simulink model "RBFNN_1221"  (R2018a)
settings: Solver=FixedStepAuto  StartTime=0.0  StopTime=inf  FixedStep=0.001  RelTol=1e-3  EnableMultiTasking=on
undefined symbols (not defined in the file): HIL, j, qc_get_step_size
libraries: dsparch4 x28, quarc_library x17, simulink x7, vrlib x1
(part 5 of 6)

== matlab function RBFNN_1221/DIARC_new ==
  data: U output; mode_IARC input; switch_NN input; RBFNN input; qd input; qd_dot input; qd_ddot input; qd_dddot input; q input; q_dot input; P_i input; P_o input; P_s input; P_r input; K_1 input; K_2 input; K_3 input; w2 input; w3 input; gamma_d1 input; gamma_d2 input; vartheta_s1 input; vartheta_s2 input; d1hat input; d2hat input; Gamma1_1 input; Gamma1_2 input; Gamma1_3 input; Gamma1_4 input; Gamma2 input; X1_f input; q_ddot input; e2 output; e3 output; vartheta_s1_next output; vartheta_s2_next output; d1hat_next output; d2hat_next output; Gamma1_1_next output; Gamma1_2_next output; Gamma1_3_next output; Gamma1_4_next output; Gamma2_next output; X1f_next output; tolook_FLd output; tolook_QLd output; tolook_others output; tolook_FLda1_joint3 output
function [U, e2, e3, vartheta_s1_next, vartheta_s2_next, d1hat_next, d2hat_next,...
    Gamma1_1_next, Gamma1_2_next, Gamma1_3_next, Gamma1_4_next, Gamma2_next, X1f_next, ...
    tolook_FLd, tolook_QLd, tolook_others,tolook_FLda1_joint3] ...
    = DIARC_new(mode_IARC, switch_NN, RBFNN, qd, qd_dot, qd_ddot, qd_dddot, q, q_dot,...
    P_i, P_o, P_s, P_r, K_1, K_2, K_3, w2, w3, gamma_d1, gamma_d2,...
    vartheta_s1, vartheta_s2, d1hat, d2hat, Gamma1_1, Gamma1_2, Gamma1_3, Gamma1_4, Gamma2, X1_f,  q_ddot)
% --------------------------程序说明---------------------------
%
% Aunthor: Yangxiu Xia
% multi-DOF 关节空间主控程序，1.0版本完成时间
%
% --------------------------输入参数---------------------------
%
%      传感器部分
% qd:           R4*1，弧度制rad，分别为J1-J4的四个期望角度
% qd_dot:       R4*1，弧度制rad，分别为J1-J4的四个期望角速度
% qd_ddot:      R4*1，弧度制rad，分别为J1-J4的四个期望角加速度
% qd_dddot:     R4*1，弧度制rad，分别为J1-J4的四个期望角加加速度
% q:            R4*1，弧度制rad，分别为J1-J4的四个实际角度
% q_dot:        R4*1，弧度制rad，分别为J1-J4的四个实际角速度，通过前置快速微分滤波得到
% P_i:          R4*1，Pa，无杆腔压力
% P_o:          R4*1，Pa，有杆腔压力
% P_s:          R1*1，Pa，泵出压力
% P_r:          R1*1，Pa，油箱参考压力
%       控制部分
% K_1:          R4*1，(使用时是diag形式)，滑模增益，
% K_2:          R4*1，(使用时是diag形式)，step1线性反馈增益
% K_3:          R4*1，(使用时是diag形式)，step2线性反馈增益
% w2:           R4*1，(使用时是diag形式)，量纲平衡系数2
% w3:           R4*1，(使用时是diag形式)，量纲平衡系数336.
% gamma_d1:     R4*1，(使用时是diag形式)，step1快速动力学补偿项的更新增益
% gamma_d2:     R4*1，(使用时是diag形式)，step2快速动力学补偿项的更新增益
% vartheta_s1:  R12*1，[f_v, f_c, D_Fn] = [4个关节的粘性摩擦, 4个关节的库伦摩擦, 4个关节的建模误差名义值]
% vartheta_s2:  R9*1， [D_Qin, D_Qon, 1/Beta_e] = [4个关节的建模误差名义值1, 4个关节的建模误差名义值2，油液弹性模量]
% d1hat:        R4*1，step1快速动力学补偿项
% d2hat:        R4*1，step2快速动力学补偿项
% Gamma1:       R12*12，自适应律增益矩阵1
% Gamma2:       R9*9，  自适应律增益矩阵2
% X_f:          R37*1,  滤波中间量 = [vartheta_s1(12，无mL), u_s1f_A(4), pF(4), vartheta_s2(9), u_s2(4), pQ(4)]
% 
% --------------------------变量维度---------------------------
%
% M0:           R4*4，（不考虑负载）机械臂本体的惯性矩阵
% C0:           R4*4，（不考虑负载）机械臂本体的离心力与科氏力矩阵
% G0:           R4*1，（不考虑负载）机械臂本体的重力矩阵
% ML:           R4*4，负载带来的额外惯性矩阵
% CL:           R4*4，负载带来的额外离心力与科氏力矩阵
% GL:           R4*1，负载带来的额外重力矩阵
% alpha_DH:     R4*1，弧度制rad，控制三角形夹角
% q_ddot:       R4*1，弧度制rad，分别为J1-J4的四个实际角加速度
% q_dddot:      R4*1，弧度制rad，分别为J1-J4的四个实际角加加速度
% tau:          R4*1，机械臂驱动力矩，包括液压缸推力与摩擦
% D_Fn:         R4*1，机械臂刚体动力学的集总建模误差名义值
% D_Qin:        R4*1，容腔压力动力学的集总建模误差1名义值
% D_Qon:        R4*1，容腔压力动力学的集总建模误差2名义值
% J_h:          R4*4，非奇异关节雅各比矩阵
% F_L:          R4*1，液压缸输出推力
% T_f:          R4*1，摩擦力矩
% f_v:          R4*1，粘性摩擦系数 
% f_c:          R4*1，库伦摩擦系数
% A_o:          R4*4，有杆腔活塞面积
% V_i:          R4*4，无杆腔可压缩容积
% V_o:          R4*4，有杆腔可压缩容积
% x_L:          R4*1，液压缸位移
% Beta_e:       R1*1，油液弹性膜模量
% Q_i:          R4*1，无杆腔供应流量
% Q_o:          R4*1，有杆腔供应流量
% K_qi:         R4*1，无杆腔阀口流量增益系数
% K_qo:         R4*1，有杆腔阀口流量增益系数
% h_i:          R4*1，无杆腔压差
% A_i:          R4*4，无杆腔活塞面积
% h_o:          R4*1，有杆腔压差
% 
% -------------------------------------------------------------

%%
%-------输入模拟（维度范例）--------
% mode_mL = 1;
% qd = [1 2 3 4]'/57;
% qd_dot = [1 2 3 4]'/57;
% qd_ddot = [1 2 3 4]'/57;
% qd_dddot = [1 2 3 4]'/57;
% q = [1 2 3 4]'/57;
% q_dot = [1 2 3 4]'/57;
% P_i = [1 2 3 4]';
% P_o = [1 2 3 4]';
% P_s = 6;
% P_r = 0;
% K_1 = [80 80 80 80]';
% K_2 = [80 80 80 80]';
% K_3 = [80 80 80 80]';
% w2 = [1 1 1 1]';
% w3 = [1 1 1 1]';
% gamma_d1 = [1 1 1 1]';
% gamma_d2 = [1 1 1 1]';
% vartheta_s1 = 1 * ones(12 ,1);
% vartheta_s2 = 1 * ones(9 ,1);
% mL_in = 0;
% d1hat = [1 1 1 1]';
% d2hat = [1 1 1 1]';
% Gamma1_1 = 1 * ones(3, 3);
% Gamma1_2 = 1 * ones(3, 3);
% Gamma1_3 = 1 * ones(3, 3);
% Gamma1_4 = 1 * ones(3, 3);
% Gamma2 = 1 * ones(9, 9);
% Gamma_mL = 1;
% X1_f = 1.0 * ones(37 ,1);
% X2_f = 1.0 * ones(16 ,1);


% 仿真环境
ts = 0.001;                                                                 % 仿真步长

% 变量预处理
theta_hat1 = vartheta_s1(1:4);                                              % 粘性摩擦系数  fv
theta_hat2 = vartheta_s1(5:8);                                              % 库伦摩擦系数  fc
theta_hat3 = vartheta_s1(9:12);                                             % 集总建模误差1 D_Fn
theta_hat4 = vartheta_s2(1:4);                                              % 集总建模误差2 D_Qin
theta_hat5 = vartheta_s2(5:8);                                              % 集总建模误差3 D_Qon
theta_hat6 = vartheta_s2(9);                                                % 油液弹性模量  1/beta_e




%-------其余默认控制器参数--------
k1 = diag(K_1);
k2 = diag(K_2);
k3 = diag(K_3);
v1 = 0.1;                                                                   % Gamma更新中的比例因子
v2 = 0.1;
alpha1 = 0.02*10;                                                              % Gamma更新中的遗忘因子 
alpha2 = 0.02*5;
tau_f = 0.006;                                                              % 一阶微分滤波时选用的时间常数
omega = diag(w2 ./ w3);                                                     % Backstepping中两次Setp的权重比

% f_v_min = 0 * ones(4, 1);
% f_c_min = 0 * ones(4, 1);
% D_Fn_min = -1e4 * ones(4, 1);

% f_v_max = 100 * ones(4, 1);
% f_c_max = 100 * ones(4, 1);
% D_Fn_max = -D_Fn_min;

vartheta_F_min = [-1e3, -150, -1e4]';
vartheta_F_max = [1e3, 1e3, 1e4]';

% vartheta_s1_min = [f_v_min', f_c_min', D_Fn_min', m_L_min]';
% vartheta_s1_max = [f_v_max', f_c_max', D_Fn_max', m_L_max]';

D_Qin_min = -1e-5 * ones(4, 1)*100*100;
D_Qin_max = -D_Qin_min;
D_Qon_min = D_Qin_min;
D_Qon_max = D_Qin_max;
Beta_e_min = 1/1e8/10;
Beta_e_max = 1/1e8*1.5;
vartheta_s2_min = [D_Qin_min', D_Qon_min', Beta_e_max]';
vartheta_s2_max = [D_Qin_max', D_Qon_max', Beta_e_min]';

Gamma1_fv_max = 1000;
Gamma1_fc_max = 250;
Gamma1_DFn_max = 100;
Gamma1_fv_min = -3000;
Gamma1_fc_min = -10;
Gamma1_DFn_min = -100;
Gamma1_max = [Gamma1_fv_max', Gamma1_fc_max', Gamma1_DFn_max']';
Gamma1_min = [Gamma1_fv_min', Gamma1_fc_min', Gamma1_DFn_min']';

Gamma2_D_Qin_max = 1e-3 * ones(4, 1);
Gamma2_D_Qon_max = Gamma2_D_Qin_max;
Gamma2_Beta_e_max = 0.1;
Gamma2_D_Qin_min = -Gamma2_D_Qin_max;
Gamma2_D_Qon_min = -Gamma2_D_Qin_max;
Gamma2_Beta_e_min = -Gamma2_Beta_e_max;
Gamma2_max = [Gamma2_D_Qin_max', Gamma2_D_Qon_max', Gamma2_Beta_e_max]';
Gamma2_min = [Gamma2_D_Qin_min', Gamma2_D_Qon_min', Gamma2_Beta_e_min]';


% ----------------------硬件参数----------------------
deg2rad = 2*pi/360;                                                         % 角度制转弧度制
mm2m = 1e-3;                                                                % 毫米制转米制
g = 9.8;                                                                    % 重力加速度
AB = [230, 261, 245, 195]' .* mm2m;                                          % 控制三角形的临边长1
BC = [46,  60,  50,  40 ]' .* mm2m;                                          % 控制三角形的临边长2

x0Total = [190, 207, 202, 162]' .* mm2m;                                    % 液压缸的初始长度（x=0）
D1 = [32, 50, 40, 32]' .* mm2m;                                             % 液压缸直径
D2 = [16, 25, 16, 16]' .* mm2m;                                             % 液压缸伸出杆直径
xmax = [80, 104, 82, 62]' .* 1e-3;                                          % 液压缸总行程长度
length1_pipeline = [500, 500+300, 500+300+100, 500+300+100+200]' .* mm2m;   % 无杆腔油管长度
length2_pipeline = [600, 600+200, 600+200+400, 600+200+400+250]' .* mm2m;   % 有杆腔油管长度
D_pipeline = 1/6 * 0.0254;                                                  % 油管直径


m = [3, 14, 4, 10];                                                   % 连杆质量（瞎估的，不准确）
L = [101.1, 605, 284.4, 484.4]' .* mm2m;                                    % 连杆长度
r = [50, 300, 140, 300]' .* mm2m;                                                                    % 连杆质心位置
Ix = [13826,  14322,  19924,  22077]' .* mm2m .* mm2m;                      % 连杆转动惯量（沿X轴方向，即沿杆子的方向的轴）
Iy = [30072, 1614730, 138744, 693699]' .* mm2m .* mm2m;                     % 连杆转动惯量（沿Y轴方向，按照关节的DH坐标轴）
Iz = [21003, 1609974, 144768, 691256]' .* mm2m .* mm2m;                     % 连杆转动惯量（沿Z轴方向，按照关节的DH坐标轴，Z轴是我们主要考虑的）
% q = [0,10/57,60/57,40/57];                                                % 连杆速度
% qd = [0,0,0.1,1];                                                         % 连杆角速度
Ix2 = Ix(2); Ix3 = Ix(3); Ix4 = Ix(4);
Iy2 = Iy(2); Iy3 = Iy(3); Iy4 = Iy(4);
Iz1 = Iz(1); Iz2 = Iz(2); Iz3 = Iz(3); Iz4 = Iz(4);
m1 = m(1); m2 = m(2); m3 = m(3); m4 = m(4);
r1 = r(1); r2 = r(2); r3 = r(3); r4 = r(4);
L1 = L(1); L2 = L(2); L3 = L(3); L4 = L(4);

% DCARC，用于控制设计
q_u = qd;
qu_dot = qd_dot;

q2 = q_u(2); q3 = q_u(3); q4 = q_u(4);
q1d = qu_dot(1); q2d = qu_dot(2); q3d = qu_dot(3); q4d = qu_dot(4);

M_0d = [Ix2/2 + Ix3/2 + Ix4/2 + Iy2/2 + Iy3/2 + Iy4/2 + Iz1 - (Ix3*cos(2*q2 + 2*q3))/2 + (Iy3*cos(2*q2 + 2*q3))/2 + L1^2*m2 + L1^2*m3 + L1^2*m4 + (L2^2*m3)/2 + (L2^2*m4)/2 + (L3^2*m3)/2 + (L3^2*m4)/2 + m1*r1^2 + (m2*r2^2)/2 + (m4*r4^2)/2 - (Ix2*cos(2*q2))/2 + (Iy2*cos(2*q2))/2 - (Ix4*cos(2*q2 + 2*q3 + 2*q4))/2 + (Iy4*cos(2*q2 + 2*q3 + 2*q4))/2 + (L2^2*m3*cos(2*q2))/2 + (L2^2*m4*cos(2*q2))/2 + (m2*r2^2*cos(2*q2))/2 + (m4*r4^2*cos(2*q2 + 2*q3 + 2*q4))/2 + (L3^2*m3*cos(2*q2 + 2*q3))/2 + (L3^2*m4*cos(2*q2 + 2*q3))/2 + 2*L1*L3*m3*cos(q2 + q3) + 2*L1*L3*m4*cos(q2 + q3) + L2*m4*r4*cos(q3 + q4) + 2*L1*L2*m3*cos(q2) + 2*L1*L2*m4*cos(q2) + L2*L3*m3*cos(q3) + L2*L3*m4*cos(q3) + 2*L1*m2*r2*cos(q2) + L3*m4*r4*cos(q4) + L3*m4*r4*cos(2*q2 + 2*q3 + q4) + L2*L3*m3*cos(2*q2 + q3) + L2*L3*m4*cos(2*q2 + q3) + 2*L1*m4*r4*cos(q2 + q3 + q4) + L2*m4*r4*cos(2*q2 + q3 + q4), 0,  0,  0;
      0, Iz2 + Iz3 + Iz4 + L2^2*m3 + L2^2*m4 + L3^2*m4 + m2*r2^2 + m3*r3^2 + m4*r4^2 + 2*L2*m4*r4*cos(q3 + q4) + 2*L2*L3*m4*cos(q3) + 2*L2*m3*r3*cos(q3) + 2*L3*m4*r4*cos(q4), m4*L3^2 + 2*m4*cos(q4)*L3*r4 + L2*m4*cos(q3)*L3 + m3*r3^2 + L2*m3*cos(q3)*r3 + m4*r4^2 + L2*m4*cos(q3 + q4)*r4 + Iz3 + Iz4, Iz4 + m4*r4^2 + L2*m4*r4*cos(q3 + q4) + L3*m4*r4*cos(q4);
      0, m4*L3^2 + 2*m4*cos(q4)*L3*r4 + L2*m4*cos(q3)*L3 + m3*r3^2 + L2*m3*cos(q3)*r3 + m4*r4^2 + L2*m4*cos(q3 + q4)*r4 + Iz3 + Iz4,     m4*L3^2 + 2*m4*cos(q4)*L3*r4 + m3*r3^2 + m4*r4^2 + Iz3 + Iz4,      m4*r4^2 + L3*m4*cos(q4)*r4 + Iz4;
      0, Iz4 + m4*r4^2 + L2*m4*r4*cos(q3 + q4) + L3*m4*r4*cos(q4),  m4*r4^2 + L3*m4*cos(q4)*r4 + Iz4,    m4*r4^2 + Iz4];
 
C_0d = [(Ix2*q2d*sin(2*q2))/2 - (Iy2*q2d*sin(2*q2))/2 + (Ix4*q2d*sin(2*q2 + 2*q3 + 2*q4))/2 + (Ix4*q3d*sin(2*q2 + 2*q3 + 2*q4))/2 + (Ix4*q4d*sin(2*q2 + 2*q3 + 2*q4))/2 - (Iy4*q2d*sin(2*q2 + 2*q3 + 2*q4))/2 - (Iy4*q3d*sin(2*q2 + 2*q3 + 2*q4))/2 - (Iy4*q4d*sin(2*q2 + 2*q3 + 2*q4))/2 + (Ix3*q2d*sin(2*q2 + 2*q3))/2 + (Ix3*q3d*sin(2*q2 + 2*q3))/2 - (Iy3*q2d*sin(2*q2 + 2*q3))/2 - (Iy3*q3d*sin(2*q2 + 2*q3))/2 - (L2^2*m3*q2d*sin(2*q2))/2 - (L2^2*m4*q2d*sin(2*q2))/2 - (m2*q2d*r2^2*sin(2*q2))/2 - (m4*q2d*r4^2*sin(2*q2 + 2*q3 + 2*q4))/2 - (m4*q3d*r4^2*sin(2*q2 + 2*q3 + 2*q4))/2 - (m4*q4d*r4^2*sin(2*q2 + 2*q3 + 2*q4))/2 - (L3^2*m3*q2d*sin(2*q2 + 2*q3))/2 - (L3^2*m3*q3d*sin(2*q2 + 2*q3))/2 - (L3^2*m4*q2d*sin(2*q2 + 2*q3))/2 - (L3^2*m4*q3d*sin(2*q2 + 2*q3))/2 - L1*m4*q2d*r4*sin(q2 + q3 + q4) - L1*m4*q3d*r4*sin(q2 + q3 + q4) - L1*m4*q4d*r4*sin(q2 + q3 + q4) - L2*m4*q2d*r4*sin(2*q2 + q3 + q4) - (L2*m4*q3d*r4*sin(2*q2 + q3 + q4))/2 - (L2*m4*q4d*r4*sin(2*q2 + q3 + q4))/2 - L1*L3*m3*q2d*sin(q2 + q3) - L1*L3*m3*q3d*sin(q2 + q3) - L1*L3*m4*q2d*sin(q2 + q3) - L1*L3*m4*q3d*sin(q2 + q3) - (L2*m4*q3d*r4*sin(q3 + q4))/2 - (L2*m4*q4d*r4*sin(q3 + q4))/2 - L1*L2*m3*q2d*sin(q2) - L1*L2*m4*q2d*sin(q2) - (L2*L3*m3*q3d*sin(q3))/2 - (L2*L3*m4*q3d*sin(q3))/2 - L1*m2*q2d*r2*sin(q2) - (L3*m4*q4d*r4*sin(q4))/2 - L3*m4*q2d*r4*sin(2*q2 + 2*q3 + q4) - L3*m4*q3d*r4*sin(2*q2 + 2*q3 + q4) - (L3*m4*q4d*r4*sin(2*q2 + 2*q3 + q4))/2 - L2*L3*m3*q2d*sin(2*q2 + q3) - (L2*L3*m3*q3d*sin(2*q2 + q3))/2 - L2*L3*m4*q2d*sin(2*q2 + q3) - (L2*L3*m4*q3d*sin(2*q2 + q3))/2, -q1d*((Iy3*sin(2*q2 + 2*q3))/2 - (Ix3*sin(2*q2 + 2*q3))/2 - (Ix2*sin(2*q2))/2 + (Iy2*sin(2*q2))/2 - (Ix4*sin(2*q2 + 2*q3 + 2*q4))/2 + (Iy4*sin(2*q2 + 2*q3 + 2*q4))/2 + (L2^2*m3*sin(2*q2))/2 + (L2^2*m4*sin(2*q2))/2 + (m2*r2^2*sin(2*q2))/2 + (m4*r4^2*sin(2*q2 + 2*q3 + 2*q4))/2 + (L3^2*m3*sin(2*q2 + 2*q3))/2 + (L3^2*m4*sin(2*q2 + 2*q3))/2 + L2*m4*r4*sin(2*q2 + q3 + q4) + L1*L3*m3*sin(q2 + q3) + L1*L3*m4*sin(q2 + q3) + L1*L2*m3*sin(q2) + L1*L2*m4*sin(q2) + L1*m2*r2*sin(q2) + L3*m4*r4*sin(2*q2 + 2*q3 + q4) + L2*L3*m3*sin(2*q2 + q3) + L2*L3*m4*sin(2*q2 + q3) + L1*m4*r4*sin(q2 + q3 + q4)), -q1d*((Iy3*sin(2*q2 + 2*q3))/2 - (Ix3*sin(2*q2 + 2*q3))/2 - (Ix4*sin(2*q2 + 2*q3 + 2*q4))/2 + (Iy4*sin(2*q2 + 2*q3 + 2*q4))/2 + (m4*r4^2*sin(2*q2 + 2*q3 + 2*q4))/2 + (L3^2*m3*sin(2*q2 + 2*q3))/2 + (L3^2*m4*sin(2*q2 + 2*q3))/2 + (L2*m4*r4*sin(2*q2 + q3 + q4))/2 + L1*L3*m3*sin(q2 + q3) + L1*L3*m4*sin(q2 + q3) + (L2*m4*r4*sin(q3 + q4))/2 + (L2*L3*m3*sin(q3))/2 + (L2*L3*m4*sin(q3))/2 + L3*m4*r4*sin(2*q2 + 2*q3 + q4) + (L2*L3*m3*sin(2*q2 + q3))/2 + (L2*L3*m4*sin(2*q2 + q3))/2 + L1*m4*r4*sin(q2 + q3 + q4)), -q1d*((Iy4*sin(2*q2 + 2*q3 + 2*q4))/2 - (Ix4*sin(2*q2 + 2*q3 + 2*q4))/2 + (m4*r4^2*sin(2*q2 + 2*q3 + 2*q4))/2 + (L2*m4*r4*sin(2*q2 + q3 + q4))/2 + (L2*m4*r4*sin(q3 + q4))/2 + (L3*m4*r4*sin(q4))/2 + (L3*m4*r4*sin(2*q2 + 2*q3 + q4))/2 + L1*m4*r4*sin(q2 + q3 + q4));
       q1d*((Iy3*sin(2*q2 + 2*q3))/2 - (Ix3*sin(2*q2 + 2*q3))/2 - (Ix2*sin(2*q2))/2 + (Iy2*sin(2*q2))/2 - (Ix4*sin(2*q2 + 2*q3 + 2*q4))/2 + (Iy4*sin(2*q2 + 2*q3 + 2*q4))/2 + (L2^2*m3*sin(2*q2))/2 + (L2^2*m4*sin(2*q2))/2 + (m2*r2^2*sin(2*q2))/2 + (m4*r4^2*sin(2*q2 + 2*q3 + 2*q4))/2 + (L3^2*m3*sin(2*q2 + 2*q3))/2 + (L3^2*m4*sin(2*q2 + 2*q3))/2 + L2*m4*r4*sin(2*q2 + q3 + q4) + L1*L3*m3*sin(q2 + q3) + L1*L3*m4*sin(q2 + q3) + L1*L2*m3*sin(q2) + L1*L2*m4*sin(q2) + L1*m2*r2*sin(q2) + L3*m4*r4*sin(2*q2 + 2*q3 + q4) + L2*L3*m3*sin(2*q2 + q3) + L2*L3*m4*sin(2*q2 + q3) + L1*m4*r4*sin(q2 + q3 + q4)),                                                                                                                                                                                                        - L2*q3d*(m3*r3*sin(q3) + m4*r4*sin(q3 + q4) + L3*m4*sin(q3)) - m4*q4d*r4*(L2*sin(q3 + q4) + L3*sin(q4)), - L2*q2d*(m3*r3*sin(q3) + m4*r4*sin(q3 + q4) + L3*m4*sin(q3)) - L2*q3d*(m3*r3*sin(q3) + m4*r4*sin(q3 + q4) + L3*m4*sin(q3)) - m4*q4d*r4*(L2*sin(q3 + q4) + L3*sin(q4)),                                                                                                                                                                                                                -m4*r4*(L2*sin(q3 + q4) + L3*sin(q4))*(q2d + q3d + q4d);
       q1d*((Iy3*sin(2*q2 + 2*q3))/2 - (Ix3*sin(2*q2 + 2*q3))/2 - (Ix4*sin(2*q2 + 2*q3 + 2*q4))/2 + (Iy4*sin(2*q2 + 2*q3 + 2*q4))/2 + (m4*r4^2*sin(2*q2 + 2*q3 + 2*q4))/2 + (L3^2*m3*sin(2*q2 + 2*q3))/2 + (L3^2*m4*sin(2*q2 + 2*q3))/2 + (L2*m4*r4*sin(2*q2 + q3 + q4))/2 + L1*L3*m3*sin(q2 + q3) + L1*L3*m4*sin(q2 + q3) + (L2*m4*r4*sin(q3 + q4))/2 + (L2*L3*m3*sin(q3))/2 + (L2*L3*m4*sin(q3))/2 + L3*m4*r4*sin(2*q2 + 2*q3 + q4) + (L2*L3*m3*sin(2*q2 + q3))/2 + (L2*L3*m4*sin(2*q2 + q3))/2 + L1*m4*r4*sin(q2 + q3 + q4)),                                                                                                                                                                                                                                               L2*q2d*(m3*r3*sin(q3) + m4*r4*sin(q3 + q4) + L3*m4*sin(q3)) - L3*m4*q4d*r4*sin(q4),  -L3*m4*q4d*r4*sin(q4),                                                                                                                                                                                                                                    -L3*m4*r4*sin(q4)*(q2d + q3d + q4d);
       q1d*((Iy4*sin(2*q2 + 2*q3 + 2*q4))/2 - (Ix4*sin(2*q2 + 2*q3 + 2*q4))/2 + (m4*r4^2*sin(2*q2 + 2*q3 + 2*q4))/2 + (L2*m4*r4*sin(2*q2 + q3 + q4))/2 + (L2*m4*r4*sin(q3 + q4))/2 + (L3*m4*r4*sin(q4))/2 + (L3*m4*r4*sin(2*q2 + 2*q3 + q4))/2 + L1*m4*r4*sin(q2 + q3 + q4)),                                                                                                                                                                                                                                                                                                                                                                                                                                                                                                                                                m4*r4*(L3*q2d*sin(q4) + L3*q3d*sin(q4) + L2*q2d*sin(q3 + q4)),                                                                        L3*m4*r4*sin(q4)*(q2d + q3d),  0];
 
G_0d = [  0;
g*(m2*r2*cos(q2) + m4*r4*cos(q2 + q3 + q4) + L3*m4*cos(q2 + q3) + m3*r3*cos(q2 + q3) + L2*m3*cos(q2) + L2*m4*cos(q2));
                                              L3*g*m4*cos(q2 + q3) + g*m3*r3*cos(q2 + q3) + g*m4*r4*cos(q2 + q3 + q4);
                                                                                            g*m4*r4*cos(q2 + q3 + q4)];


% IARC，用于自适应律
q_u = q;
qu_dot = q_dot;

q2 = q_u(2); q3 = q_u(3); q4 = q_u(4);
q1d = qu_dot(1); q2d = qu_dot(2); q3d = qu_dot(3); q4d = qu_dot(4);

M_0 = [Ix2/2 + Ix3/2 + Ix4/2 + Iy2/2 + Iy3/2 + Iy4/2 + Iz1 - (Ix3*cos(2*q2 + 2*q3))/2 + (Iy3*cos(2*q2 + 2*q3))/2 + L1^2*m2 + L1^2*m3 + L1^2*m4 + (L2^2*m3)/2 + (L2^2*m4)/2 + (L3^2*m3)/2 + (L3^2*m4)/2 + m1*r1^2 + (m2*r2^2)/2 + (m4*r4^2)/2 - (Ix2*cos(2*q2))/2 + (Iy2*cos(2*q2))/2 - (Ix4*cos(2*q2 + 2*q3 + 2*q4))/2 + (Iy4*cos(2*q2 + 2*q3 + 2*q4))/2 + (L2^2*m3*cos(2*q2))/2 + (L2^2*m4*cos(2*q2))/2 + (m2*r2^2*cos(2*q2))/2 + (m4*r4^2*cos(2*q2 + 2*q3 + 2*q4))/2 + (L3^2*m3*cos(2*q2 + 2*q3))/2 + (L3^2*m4*cos(2*q2 + 2*q3))/2 + 2*L1*L3*m3*cos(q2 + q3) + 2*L1*L3*m4*cos(q2 + q3) + L2*m4*r4*cos(q3 + q4) + 2*L1*L2*m3*cos(q2) + 2*L1*L2*m4*cos(q2) + L2*L3*m3*cos(q3) + L2*L3*m4*cos(q3) + 2*L1*m2*r2*cos(q2) + L3*m4*r4*cos(q4) + L3*m4*r4*cos(2*q2 + 2*q3 + q4) + L2*L3*m3*cos(2*q2 + q3) + L2*L3*m4*cos(2*q2 + q3) + 2*L1*m4*r4*cos(q2 + q3 + q4) + L2*m4*r4*cos(2*q2 + q3 + q4), 0,  0,  0;
      0, Iz2 + Iz3 + Iz4 + L2^2*m3 + L2^2*m4 + L3^2*m4 + m2*r2^2 + m3*r3^2 + m4*r4^2 + 2*L2*m4*r4*cos(q3 + q4) + 2*L2*L3*m4*cos(q3) + 2*L2*m3*r3*cos(q3) + 2*L3*m4*r4*cos(q4), m4*L3^2 + 2*m4*cos(q4)*L3*r4 + L2*m4*cos(q3)*L3 + m3*r3^2 + L2*m3*cos(q3)*r3 + m4*r4^2 + L2*m4*cos(q3 + q4)*r4 + Iz3 + Iz4, Iz4 + m4*r4^2 + L2*m4*r4*cos(q3 + q4) + L3*m4*r4*cos(q4);
      0, m4*L3^2 + 2*m4*cos(q4)*L3*r4 + L2*m4*cos(q3)*L3 + m3*r3^2 + L2*m3*cos(q3)*r3 + m4*r4^2 + L2*m4*cos(q3 + q4)*r4 + Iz3 + Iz4,     m4*L3^2 + 2*m4*cos(q4)*L3*r4 + m3*r3^2 + m4*r4^2 + Iz3 + Iz4,      m4*r4^2 + L3*m4*cos(q4)*r4 + Iz4;
      0, Iz4 + m4*r4^2 + L2*m4*r4*cos(q3 + q4) + L3*m4*r4*cos(q4),  m4*r4^2 + L3*m4*cos(q4)*r4 + Iz4,    m4*r4^2 + Iz4];
 
C_0 = [(Ix2*q2d*sin(2*q2))/2 - (Iy2*q2d*sin(2*q2))/2 + (Ix4*q2d*sin(2*q2 + 2*q3 + 2*q4))/2 + (Ix4*q3d*sin(2*q2 + 2*q3 + 2*q4))/2 + (Ix4*q4d*sin(2*q2 + 2*q3 + 2*q4))/2 - (Iy4*q2d*sin(2*q2 + 2*q3 + 2*q4))/2 - (Iy4*q3d*sin(2*q2 + 2*q3 + 2*q4))/2 - (Iy4*q4d*sin(2*q2 + 2*q3 + 2*q4))/2 + (Ix3*q2d*sin(2*q2 + 2*q3))/2 + (Ix3*q3d*sin(2*q2 + 2*q3))/2 - (Iy3*q2d*sin(2*q2 + 2*q3))/2 - (Iy3*q3d*sin(2*q2 + 2*q3))/2 - (L2^2*m3*q2d*sin(2*q2))/2 - (L2^2*m4*q2d*sin(2*q2))/2 - (m2*q2d*r2^2*sin(2*q2))/2 - (m4*q2d*r4^2*sin(2*q2 + 2*q3 + 2*q4))/2 - (m4*q3d*r4^2*sin(2*q2 + 2*q3 + 2*q4))/2 - (m4*q4d*r4^2*sin(2*q2 + 2*q3 + 2*q4))/2 - (L3^2*m3*q2d*sin(2*q2 + 2*q3))/2 - (L3^2*m3*q3d*sin(2*q2 + 2*q3))/2 - (L3^2*m4*q2d*sin(2*q2 + 2*q3))/2 - (L3^2*m4*q3d*sin(2*q2 + 2*q3))/2 - L1*m4*q2d*r4*sin(q2 + q3 + q4) - L1*m4*q3d*r4*sin(q2 + q3 + q4) - L1*m4*q4d*r4*sin(q2 + q3 + q4) - L2*m4*q2d*r4*sin(2*q2 + q3 + q4) - (L2*m4*q3d*r4*sin(2*q2 + q3 + q4))/2 - (L2*m4*q4d*r4*sin(2*q2 + q3 + q4))/2 - L1*L3*m3*q2d*sin(q2 + q3) - L1*L3*m3*q3d*sin(q2 + q3) - L1*L3*m4*q2d*sin(q2 + q3) - L1*L3*m4*q3d*sin(q2 + q3) - (L2*m4*q3d*r4*sin(q3 + q4))/2 - (L2*m4*q4d*r4*sin(q3 + q4))/2 - L1*L2*m3*q2d*sin(q2) - L1*L2*m4*q2d*sin(q2) - (L2*L3*m3*q3d*sin(q3))/2 - (L2*L3*m4*q3d*sin(q3))/2 - L1*m2*q2d*r2*sin(q2) - (L3*m4*q4d*r4*sin(q4))/2 - L3*m4*q2d*r4*sin(2*q2 + 2*q3 + q4) - L3*m4*q3d*r4*sin(2*q2 + 2*q3 + q4) - (L3*m4*q4d*r4*sin(2*q2 + 2*q3 + q4))/2 - L2*L3*m3*q2d*sin(2*q2 + q3) - (L2*L3*m3*q3d*sin(2*q2 + q3))/2 - L2*L3*m4*q2d*sin(2*q2 + q3) - (L2*L3*m4*q3d*sin(2*q2 + q3))/2, -q1d*((Iy3*sin(2*q2 + 2*q3))/2 - (Ix3*sin(2*q2 + 2*q3))/2 - (Ix2*sin(2*q2))/2 + (Iy2*sin(2*q2))/2 - (Ix4*sin(2*q2 + 2*q3 + 2*q4))/2 + (Iy4*sin(2*q2 + 2*q3 + 2*q4))/2 + (L2^2*m3*sin(2*q2))/2 + (L2^2*m4*sin(2*q2))/2 + (m2*r2^2*sin(2*q2))/2 + (m4*r4^2*sin(2*q2 + 2*q3 + 2*q4))/2 + (L3^2*m3*sin(2*q2 + 2*q3))/2 + (L3^2*m4*sin(2*q2 + 2*q3))/2 + L2*m4*r4*sin(2*q2 + q3 + q4) + L1*L3*m3*sin(q2 + q3) + L1*L3*m4*sin(q2 + q3) + L1*L2*m3*sin(q2) + L1*L2*m4*sin(q2) + L1*m2*r2*sin(q2) + L3*m4*r4*sin(2*q2 + 2*q3 + q4) + L2*L3*m3*sin(2*q2 + q3) + L2*L3*m4*sin(2*q2 + q3) + L1*m4*r4*sin(q2 + q3 + q4)), -q1d*((Iy3*sin(2*q2 + 2*q3))/2 - (Ix3*sin(2*q2 + 2*q3))/2 - (Ix4*sin(2*q2 + 2*q3 + 2*q4))/2 + (Iy4*sin(2*q2 + 2*q3 + 2*q4))/2 + (m4*r4^2*sin(2*q2 + 2*q3 + 2*q4))/2 + (L3^2*m3*sin(2*q2 + 2*q3))/2 + (L3^2*m4*sin(2*q2 + 2*q3))/2 + (L2*m4*r4*sin(2*q2 + q3 + q4))/2 + L1*L3*m3*sin(q2 + q3) + L1*L3*m4*sin(q2 + q3) + (L2*m4*r4*sin(q3 + q4))/2 + (L2*L3*m3*sin(q3))/2 + (L2*L3*m4*sin(q3))/2 + L3*m4*r4*sin(2*q2 + 2*q3 + q4) + (L2*L3*m3*sin(2*q2 + q3))/2 + (L2*L3*m4*sin(2*q2 + q3))/2 + L1*m4*r4*sin(q2 + q3 + q4)), -q1d*((Iy4*sin(2*q2 + 2*q3 + 2*q4))/2 - (Ix4*sin(2*q2 + 2*q3 + 2*q4))/2 + (m4*r4^2*sin(2*q2 + 2*q3 + 2*q4))/2 + (L2*m4*r4*sin(2*q2 + q3 + q4))/2 + (L2*m4*r4*sin(q3 + q4))/2 + (L3*m4*r4*sin(q4))/2 + (L3*m4*r4*sin(2*q2 + 2*q3 + q4))/2 + L1*m4*r4*sin(q2 + q3 + q4));
       q1d*((Iy3*sin(2*q2 + 2*q3))/2 - (Ix3*sin(2*q2 + 2*q3))/2 - (Ix2*sin(2*q2))/2 + (Iy2*sin(2*q2))/2 - (Ix4*sin(2*q2 + 2*q3 + 2*q4))/2 + (Iy4*sin(2*q2 + 2*q3 + 2*q4))/2 + (L2^2*m3*sin(2*q2))/2 + (L2^2*m4*sin(2*q2))/2 + (m2*r2^2*sin(2*q2))/2 + (m4*r4^2*sin(2*q2 + 2*q3 + 2*q4))/2 + (L3^2*m3*sin(2*q2 + 2*q3))/2 + (L3^2*m4*sin(2*q2 + 2*q3))/2 + L2*m4*r4*sin(2*q2 + q3 + q4) + L1*L3*m3*sin(q2 + q3) + L1*L3*m4*sin(q2 + q3) + L1*L2*m3*sin(q2) + L1*L2*m4*sin(q2) + L1*m2*r2*sin(q2) + L3*m4*r4*sin(2*q2 + 2*q3 + q4) + L2*L3*m3*sin(2*q2 + q3) + L2*L3*m4*sin(2*q2 + q3) + L1*m4*r4*sin(q2 + q3 + q4)),                                                                                                                                                                                                        - L2*q3d*(m3*r3*sin(q3) + m4*r4*sin(q3 + q4) + L3*m4*sin(q3)) - m4*q4d*r4*(L2*sin(q3 + q4) + L3*sin(q4)), - L2*q2d*(m3*r3*sin(q3) + m4*r4*sin(q3 + q4) + L3*m4*sin(q3)) - L2*q3d*(m3*r3*sin(q3) + m4*r4*sin(q3 + q4) + L3*m4*sin(q3)) - m4*q4d*r4*(L2*sin(q3 + q4) + L3*sin(q4)),                                                                                                                                                                                                                -m4*r4*(L2*sin(q3 + q4) + L3*sin(q4))*(q2d + q3d + q4d);
       q1d*((Iy3*sin(2*q2 + 2*q3))/2 - (Ix3*sin(2*q2 + 2*q3))/2 - (Ix4*sin(2*q2 + 2*q3 + 2*q4))/2 + (Iy4*sin(2*q2 + 2*q3 + 2*q4))/2 + (m4*r4^2*sin(2*q2 + 2*q3 + 2*q4))/2 + (L3^2*m3*sin(2*q2 + 2*q3))/2 + (L3^2*m4*sin(2*q2 + 2*q3))/2 + (L2*m4*r4*sin(2*q2 + q3 + q4))/2 + L1*L3*m3*sin(q2 + q3) + L1*L3*m4*sin(q2 + q3) + (L2*m4*r4*sin(q3 + q4))/2 + (L2*L3*m3*sin(q3))/2 + (L2*L3*m4*sin(q3))/2 + L3*m4*r4*sin(2*q2 + 2*q3 + q4) + (L2*L3*m3*sin(2*q2 + q3))/2 + (L2*L3*m4*sin(2*q2 + q3))/2 + L1*m4*r4*sin(q2 + q3 + q4)),                                                                                                                                                                                                                                               L2*q2d*(m3*r3*sin(q3) + m4*r4*sin(q3 + q4) + L3*m4*sin(q3)) - L3*m4*q4d*r4*sin(q4),  -L3*m4*q4d*r4*sin(q4),                                                                                                                                                                                                                                    -L3*m4*r4*sin(q4)*(q2d + q3d + q4d);
       q1d*((Iy4*sin(2*q2 + 2*q3 + 2*q4))/2 - (Ix4*sin(2*q2 + 2*q3 + 2*q4))/2 + (m4*r4^2*sin(2*q2 + 2*q3 + 2*q4))/2 + (L2*m4*r4*sin(2*q2 + q3 + q4))/2 + (L2*m4*r4*sin(q3 + q4))/2 + (L3*m4*r4*sin(q4))/2 + (L3*m4*r4*sin(2*q2 + 2*q3 + q4))/2 + L1*m4*r4*sin(q2 + q3 + q4)),                                                                                                                                                                                                                                                                                                                                                                                                                                                                                                                                                m4*r4*(L3*q2d*sin(q4) + L3*q3d*sin(q4) + L2*q2d*sin(q3 + q4)),                                                                        L3*m4*r4*sin(q4)*(q2d + q3d),  0];
 
G_0 = [  0;
g*(m2*r2*cos(q2) + m4*r4*cos(q2 + q3 + q4) + L3*m4*cos(q2 + q3) + m3*r3*cos(q2 + q3) + L2*m3*cos(q2) + L2*m4*cos(q2));
                                              L3*g*m4*cos(q2 + q3) + g*m3*r3*cos(q2 + q3) + g*m4*r4*cos(q2 + q3 + q4);
                                                                                            g*m4*r4*cos(q2 + q3 + q4)];



% 雅各比系数
% coe_q2alpha  = [   -1,     1,      1,    -1]';                              % 由液压缸的放置姿态决定
coe_q2alpha  = [    -1,     1,      1,     -1]';                              % 由液压缸的放置姿态决定
bias_q2alpha = [-84.24, 52.96, 188.35, -64.18]' .* deg2rad;
alpha_DH = coe_q2alpha .* q + bias_q2alpha;
alpha_d_DH = coe_q2alpha .* qd + bias_q2alpha;
xNowTotal = ones(4, 1);
xNowTotal_d = ones(4, 1);
for ii = 1:4
  xNowTotal(ii) = sqrt(AB(ii)^2 + BC(ii)^2 - 2*AB(ii)*BC(ii)*cos(alpha_DH(ii)));           	% 控制三角形中关节角对应的边长
  xNowTotal_d(ii) = sqrt(AB(ii)^2 + BC(ii)^2 - 2*AB(ii)*BC(ii)*cos(alpha_d_DH(ii)));           	% 控制三角形中关节角对应的边长
end
sign1 = [-1, 1, 1, -1]';
J_h = diag(sign1) * diag((AB .* BC .* sin(alpha_DH)) ./ xNowTotal);
inv_J_h = diag(sign1) * diag(xNowTotal ./ (AB .* BC .* sin(alpha_DH)));
Jd_h = diag(sign1) * diag((AB .* BC .* sin(alpha_d_DH)) ./ xNowTotal_d);
inv_Jd_h = diag(sign1) * diag(xNowTotal_d ./ (AB .* BC .* sin(alpha_d_DH)));

% 液压相关
A_pipeline = 0.25*pi*D_pipeline^2;                                          % R1*1, 油管面积
Ai = diag(0.25*pi*D1.^2);                                                   % R4*4, 无杆腔面积
Ao = Ai - diag(0.25*pi*D2.^2);                                              % R4*4, 有杆腔面积
Vh1 = A_pipeline * length1_pipeline;                                        % R4*1, 无杆腔油管油液体积
Vh2 = A_pipeline * length2_pipeline + Ao*xmax;                              % R4*1, 有杆腔油管油液体积
xL = xNowTotal - x0Total;                                                   % R4*1, 液压缸位移
Vi = diag(Vh1 + Ai * xL);                                                   % R4*4, 无杆腔油液总体积
Vo = diag(Vh2 - Ao * xL);                                                   % R4*4, 有杆腔油液总体积


% F_L = coe_q2alpha .* (Ai*P_i - Ao*P_o);
% 大臂油缸反向布置
% coe_FL = [    1,     -1,      1,     1]';
% coe_FL = [    1,     -1,      -1,     -1]';
F_L = (Ai*P_i - Ao*P_o);

%-------DIARC Controller Design--------
% 控制目标预处理
e1 = q - qd;                                                                % 角度跟踪误差
e1_dot = q_dot - qd_dot;
q_eq_dot = qd_dot - k1*e1;                                                  % 等效跟踪角速度
q_eq_ddot = qd_ddot - k1*e1_dot;
e2 = q_dot - q_eq_dot;                                                      % 类滑模量
% step 1
S_qdot = 2/pi*atan(900*q_dot);                                           % 库仑摩擦力的近似，以保证连续可导，值域(-1,1)
Sd_qdot = 2/pi*atan(900*qd_dot);
Tf_hat = diag(q_dot)*theta_hat1 + diag(S_qdot)*theta_hat2;
Tfd_hat = diag(qd_dot)*theta_hat1 + diag(Sd_qdot)*theta_hat2;

% FLda1 = inv_J_h * (M_0d*q_eq_ddot + C_0d*q_eq_dot + G_0d + (M_Ld*q_eq_ddot + C_Ld*q_eq_dot + G_Ld)*mL_hat + Tf_hat - theta_hat3);
FLda1 = inv_Jd_h * (M_0d*qd_ddot + C_0d*qd_dot + G_0d + Tfd_hat - theta_hat3);%?????
% FLda1 = inv_J_h * (M_0d*q_eq_ddot + C_0d*q_eq_dot + G_0d + Tfd_hat - theta_hat3);
FLda2 = -inv_J_h * d1hat .* 1;
FLdNN = [0; 0; -RBFNN(3) * switch_NN; -RBFNN(1) * switch_NN;];
FLds1 = -inv_J_h * k2 * e2;                                                 % 线性稳定反馈项
FLds2 = 0;                                                                  % 非线性稳定反馈项（很小，暂不设计）;
FLd = FLda1 + FLda2 + FLds1 + FLdNN;
%FLd = FLds1;                                                               %%%%%%%%%%%%%%%%%%%%%%
% 中间项计算
% pFLdpq = - 1/pxpq * k2s1 * k1 * Alpha;
% pFLdpq = - 1/J_h * k2s1 * k1 * ThetaHat(1);                                % 2022.04.08更新，原来的这两项求错了
% % pFLdpqdot = 1/pxpq*ThetaHat(2) + pxpq*ThetaHat(3) - 1/pxpq*k2s1;
% pFLdpqdot = J_h*ThetaHat(2) + 1/J_h*ThetaHat(3) - 1/J_h*k2s1*ThetaHat(1) - 1/J_h*ThetaHat(1)*k1; % 2022.04.08更新
% pFLdpt = 1/J_h*(AlphaHopedddot+k1*AlphaHopeddot)*ThetaHat(1) + 1/J_h*k2s1*ThetaHat(1)*(AlphaHopeddot+k1*AlphaHopedot);
% AlphaddotHat = 1/ThetaHat(1)*(J_h*F_L - J_h^2*Alphadot*ThetaHat(2) - Alphadot*ThetaHat(3) - J_h*Sf1*ThetaHat(4) - Sf2*ThetaHat(5) + ThetaHat(6));
% FLdc_dot = pFLdpq*Alphadot + pFLdpqdot*AlphaddotHat + pFLdpt;             % 虚拟控制力的微分的可计算部分
FLdc_dot = 0 * ones(4, 1);

% step 2
% 简记
A_Q = Ai^2/Vi + Ao^2/Vo;
B_Q = Ai / Vi;
C_Q = Ao / Vo;

Upsilon_Q = -J_h * omega * e2;                                              % Backstepping中需要的补偿项，其作用在李雅普诺夫稳定性证明中体现
% Upsilon_Q = 0;                                                              %%%%%%%%%%%%%%%%%%%%%%%%%
% 计算
e3 = F_L - FLd;
% QLda1 = J_h*A_Q*q_dot - B_Q*theta_hat4 - C_Q*theta_hat5 + FLdc_dot*theta_hat6 + Upsilon_Q;
QLda1 = Jd_h*A_Q*qd_dot - B_Q*theta_hat4 - C_Q*theta_hat5 + FLdc_dot*theta_hat6;
QLda2 = -d2hat .* 1;
QLdNN = [0; 0;  -RBFNN(4) * switch_NN; -RBFNN(2) * switch_NN;];
QLda4 = Upsilon_Q;
QLds1 = -k3 * vartheta_s2_max(9) * e3;                                           %%%%%%%%%%%%%%%%%%%%%%%%%%%%%%%%%%%%%%%%%%%%%
QLd = QLda1 + QLda2 + QLdNN + QLda4 + QLds1;
QLd_use = QLd;
% QLd = QLds1;

%% ----------------------滤波处理----------------------
% 空载状态
temp0 = zeros(37, 1);  

A_org = J_h*F_L + C_0'*q_dot - G_0;
B_org = M_0*q_dot;
C_org = q_dot;
D_org = S_qdot;
E_org = -ones(4, 1);
temp0(1:20) = [A_org', B_org', C_org', D_org', E_org'];

phi2 = [diag(B_Q); diag(C_Q); 0];                                           % R9*1, 对于矩阵A而言，diag(A)=提取主对角线元素
us2f = QLd - J_h*A_Q*q_dot;                                                 % R4*1
pQ = F_L;                                                                   % R4*1
temp0(21:29) = phi2;
temp0(30:33) = us2f;
temp0(34:37) = pQ;

% Xf_next = zeros(37, 1);  
X1f_next = (temp0 - X1_f) ./ tau_f .* ts + X1_f;                               % 一阶微分滤波
%（注意：此处只是更新了Xf，但是pF和pQ需要通过一阶微分额外得到实际需要的导数值）

% 将滤波后的值给到线性回归矩阵与对应的输入（用作后续最小二乘的参数自适应）
A_f = X1f_next(1:4);
B_f = (temp0(5:8) - X1_f(5: 8)) ./ tau_f;
C_f = X1f_next(9:12);
D_f = X1f_next(13:16);
E_f = X1f_next(17:20);

u1f_phi = B_f - A_f;
phi1f_bar_1 = [C_f(1), D_f(1), E_f(1)]';  %列向量
phi1f_bar_2 = [C_f(2), D_f(2), E_f(2)]';  %列向量
phi1f_bar_3 = [C_f(3), D_f(3), E_f(3)]';  %列向量
phi1f_bar_4 = [C_f(4), D_f(4), E_f(4)]';  %列向量
u1f_phi_1 = u1f_phi(1);
u1f_phi_2 = u1f_phi(2);
u1f_phi_3 = u1f_phi(3);
u1f_phi_4 = u1f_phi(4);
vartheta_F_1 = [vartheta_s1(1), vartheta_s1(5), vartheta_s1(9)]';
vartheta_F_2 = [vartheta_s1(2), vartheta_s1(6), vartheta_s1(10)]';
vartheta_F_3 = [vartheta_s1(3), vartheta_s1(7), vartheta_s1(11)]';
vartheta_F_4 = [vartheta_s1(4), vartheta_s1(8), vartheta_s1(12)]';



% pF_dot_f = (temp0(17:20) - X1_f(17:20)) ./ tau_f;
% u1f_phi = X1f_next(13:16) - pF_dot_f;                                        % theta1-3部分的输入的滤波值
% phi1f_bar = X1f_next(1:12);                                                  % 

pQ_dot_f = (temp0(34:37) - X1_f(34:37)) ./ tau_f;
u2f_phi = X1f_next(30:33);                                                   % theta1-6部分的输入的滤波值
phi2f_bar = [diag(X1f_next(21:24)), diag(X1f_next(25:28)), pQ_dot_f]';

% 压力动力学参数自适应
Gamma1_1_next = Gamma1_1;
Gamma1_2_next = Gamma1_2;
Gamma1_3_next = Gamma1_3;
Gamma1_4_next = Gamma1_4;


% 程序完备性
vartheta_F_1_next = vartheta_F_1;
vartheta_F_2_next = vartheta_F_2;
vartheta_F_3_next = vartheta_F_3;
vartheta_F_4_next = vartheta_F_4;
for idx_joint = 1:4
    % 数据传入
    switch idx_joint
        case 1
            phi1f_bar_in = phi1f_bar_1;
            vartheta_F_in = vartheta_F_1;
            u1f_phi_in = u1f_phi_1;
            Gamma_in = Gamma1_1;
        case 2
            phi1f_bar_in = phi1f_bar_2;
            vartheta_F_in = vartheta_F_2;
            u1f_phi_in = u1f_phi_2;
            Gamma_in = Gamma1_2;
        case 3
            phi1f_bar_in = phi1f_bar_3;
            vartheta_F_in = vartheta_F_3;
            u1f_phi_in = u1f_phi_3;
            Gamma_in = Gamma1_3;
        case 4
            phi1f_bar_in = phi1f_bar_4;
            vartheta_F_in = vartheta_F_4;
            u1f_phi_in = u1f_phi_4;
            Gamma_in = Gamma1_4;
        otherwise
            phi1f_bar_in = zeros(3, 1);
            vartheta_F_in = zeros(3, 1);
            u1f_phi_in = zeros(1, 1);
            Gamma_in = zeros(3, 3);
    end

    Epsilon_in = -phi1f_bar_in' * vartheta_F_in - u1f_phi_in;                          % Epsilon_1代表预估误差（thetahat默认是列向量） R_1*1
    xi_in = 1 / (1+v1*(phi1f_bar_in')*Gamma_in*phi1f_bar_in);                            % 为书写方便，简记 R_1*1
    tau_in = xi_in * phi1f_bar_in * Epsilon_in;                                        % 自适应函数1 R_6*1
    vartheta_F_in_dot = Gamma_in * tau_in;
    vartheta_F_in_next = vartheta_F_in + vartheta_F_in_dot*ts;
    for idx_upd = 1:3
        if( vartheta_F_in_next(idx_upd)>vartheta_F_min(idx_upd) ) && (vartheta_F_in_next(idx_upd)<vartheta_F_max(idx_upd))
        else
            vartheta_F_in_next = vartheta_F_in;
        end
    end
    Gamma_in_dot = alpha1*Gamma_in - xi_in*Gamma_in*phi1f_bar_in*(phi1f_bar_in')*Gamma_in;
    Gamma_in_next = Gamma_in_dot*ts + Gamma_in;
    for idx_gi = 1:3
        for idx_gj = 1:3
            if Gamma_in_next(idx_gi,idx_gj) > Gamma1_max(idx_gi)
                Gamma_in_next(idx_gi,idx_gj) = Gamma1_max(idx_gi);
            end
            if Gamma_in_next(idx_gi,idx_gj) < Gamma1_min(idx_gi)
                Gamma_in_next(idx_gi,idx_gj) = Gamma1_min(idx_gi);
            end
        end
    end

    % 数据输出
    switch idx_joint
        case 1
            vartheta_F_1_next = vartheta_F_in_next;
            Gamma1_1_next = Gamma_in_next;
        case 2
            vartheta_F_2_next = vartheta_F_in_next;
            Gamma1_2_next = Gamma_in_next;
        case 3
            vartheta_F_3_next = vartheta_F_in_next;
            Gamma1_3_next = Gamma_in_next;
        case 4
            vartheta_F_4_next = vartheta_F_in_next;
            Gamma1_4_next = Gamma_in_next;
    end
end
vartheta_s1_next = vartheta_s1;
vartheta_s1_next([1 5  9]) = vartheta_F_1_next;
vartheta_s1_next([2 6 10]) = vartheta_F_2_next;
vartheta_s1_next([3 7 11]) = vartheta_F_3_next;
vartheta_s1_next([4 8 12]) = vartheta_F_4_next;


% theta 4-6
Epsilon_2 = -phi2f_bar' * vartheta_s2 - u2f_phi;
xi_2 = 1;
% xi_in = 1 / (1+v1*(phi1f_bar_in')*Gamma_in*phi1f_bar_in);
% xi_2 = 1 / (1+v2*(phi2f_bar')*Gamma2*phi2f_bar);                            % 简记
tau2 = xi_2 * phi2f_bar * Epsilon_2;
% thetahatdot_2 = 1.0*zeros(9, 1);                                            % 用于存放theta的一阶导
thetahatdot_2 = Gamma2 * tau2;

vartheta_s2_next = vartheta_s2 + thetahatdot_2*ts;
for idx_upd = 1:9
    if vartheta_s2_next(idx_upd) > vartheta_s2_max(idx_upd)
        vartheta_s2_next(idx_upd) = vartheta_s2_max(idx_upd);
    end
    if vartheta_s2_next(idx_upd) < vartheta_s2_min(idx_upd)
        vartheta_s2_next(idx_upd) = vartheta_s2_min(idx_upd);
    end
end
% Gamma2
Gamma2_dot = alpha2*Gamma2 - xi_2*Gamma2*phi2f_bar*(phi2f_bar')*Gamma2;
Gamma2_next = Gamma2_dot*ts + Gamma2;
for idx_gi = 1:9
    for idx_gj = 1:9
        if Gamma2_next(idx_gi,idx_gj) > Gamma2_max(idx_gi)
            Gamma2_next(idx_gi,idx_gj) = Gamma2_max(idx_gi);
        end
        if Gamma2_next(idx_gi,idx_gj) < Gamma2_min(idx_gi)
            Gamma2_next(idx_gi,idx_gj) = Gamma2_min(idx_gi);
        end
    end
end
% 基座是关节1 大臂是关节2 小臂是关节3 手腕是关节4
joint_index = 2;
other_joint = [1,2,3,4, 5,6,7,8, 9,10,11,12];
if mode_IARC == 0
    vartheta_s1_next(other_joint) = vartheta_s1(other_joint);
    vartheta_s2_next(other_joint) = vartheta_s2(other_joint);
end



%% ----------------------dihat更新----------------------
d1hat_dot = gamma_d1 .* e2;
d2hat_dot = gamma_d2 .* e3;
d1hat_next = d1hat_dot*ts + d1hat;
d2hat_next = d2hat_dot*ts + d2hat;

d1max = ones(4 ,1) .* 1e3;
d2max = ones(4 ,1) .* 10e-4;
d1min = -d1max;
d2min = -d2max;
for idx = 1:4
    if d1hat_next(idx) > d1max(idx)
        d1hat_next(idx) = d1max(idx);
    end
    if d1hat_next(idx) < d1min(idx)
        d1hat_next(idx) = d1min(idx);
    end

    if d2hat_next(idx) > d2max(idx)
        d2hat_next(idx) = d2max(idx);
    end
    if d2hat_next(idx) < d2min(idx)
        d2hat_next(idx) = d2min(idx);
    end
end


%% ----------------------控制输出----------------------
% Q2U
k_qi = 1.069e-9;                         	% 流量增益系数1
k_qo = 1.069e-9;                           	% 流量增益系数2
k = 10;                                    	% 电压-阀口开度映射增益

Delta_p1 = zeros(4,1);
Delta_p2 = zeros(4,1);
for ii = 1:4
    if QLd(ii) > 0 % forword
        Delta_p1(ii) = P_s - P_i(ii);
        Delta_p2(ii) = P_o(ii) - P_r;
    else % backspacings
        Delta_p1(ii) = P_i(ii) - P_r;
        Delta_p2(ii) = P_s - P_o(ii);
    end
end
coe_U = [-1, -1, -1, -1*(-1)]';%因为外部开关还有一个增益
% coe_U = [1, 1, 1, -1]';
bias_U = [0.18; 0.365; 0.18; 0.21];

Xv = QLd_use ./ (diag(B_Q).*k_qi.*sqrt(Delta_p1) + diag(C_Q).*k_qo.*sqrt(Delta_p2));
U = coe_U .* 1./k .* Xv - bias_U;                            	% 控制器输出电压

% 输出电压限幅
Umax = 10;
for idx = 1:4
    if U(idx) > Umax
        U(idx) = Umax;
    end
    if U(idx) < -Umax
        U(idx) = -Umax;
    end
end

% u = [0;0;0;0];
tolook_FLd = [FLds1; FLda1; FLda2; FLdNN];
tolook_QLd = [QLds1; QLda1; QLda2; QLdNN];
tolook_others = [FLd; QLd; inv_Jd_h(4,4); G_0d(4); g*m4*r4*cos(q2 + q3 + q4); cos(q2 + q3 + q4); e1];
tolook_FLda1_joint3 = M_0d*q_eq_ddot + C_0d*q_eq_dot + G_0d + Tfd_hat;

== matlab function RBFNN_1221/RBFNN_wrist ==
  data: W_F input; W_Q input; U_F output; U_Q output; z1 input; z2 input; W_F_next output; W_Q_next output; W_F_dot output; z3 input; p1 input; p2 input; qd input; qd_dot input; qd_ddot input; gamma_NN_F input; gamma_NN_Q input; eta_F input; eta_Q input; look output
function [U_F, U_Q, W_F_next, W_Q_next,  W_F_dot, look] = RBFNN(W_F, W_Q, z1, z2, z3, p1, p2, qd, qd_dot, qd_ddot,... 
gamma_NN_F, gamma_NN_Q, eta_F, eta_Q)

% 仿真环境
ts = 0.0002;

%-------控制器需输入信息--------

% RBFNN控制参数

%手腕关节中心点参数
%%-------
cij = [-0.850296207027729,-0.850296207027729,-1361.70740087499,4196551.85254013,2228547.18355022,0.195146877086374,0.0217376508997163,-0.106388486849609;
    -0.891195905090023,-0.891195905090023,-3679.37788134909,2763121.87654167,2209950.52011242,-0.489664101191431,-0.0473990861179181,0.146051160469149;
    -0.946370466291565,-0.946370466291565,-3684.72995146152,3042161.76989368,2145070.30294018,-0.390520008833687,-0.0780255878055779,0.337795912329846;
    -1.01730475063218,-1.01730475063218,-2819.34496924037,3432183.64498130,2145422.56092682,-0.0644644049513977,0.0210100849809342,-0.173539040975735;
    -0.744992145966297,-0.744992145966297,-1727.39328863678,3828729.80965654,2165078.72683861,0.140428689974103,0.125148334840723,-0.347091068674395;]';
cij = [-0.636278789136271,-0.636278789136271,  -2074.04256487134,4195976.19793906,2145386.16517403,0.194082222380461,0.0271921429562414,-0.120815711610908;
    -0.648723974060839,-0.648723974060839,   -5291.05357313756,2704077.74185377,2237154.84171588,-0.490879960204510,-0.0431219448842407,0.138761879553355;
    -0.613812777180803,-0.613812777180803,   -2700.03571676201,3805493.67571395,2105338.07051668,0.134104171341305,0.125264150545743,-0.359971401308276;
    -0.703512429895382,-0.703512429895382,   -5537.53448038494,2989681.25555462,2127646.48631249,-0.413038641645212,-0.0354687013635162,0.360573395246988;
    -0.798807863154537,-0.798807863154537,   -4543.22894646345,3394111.34012788,2091328.53576267,-0.0977017803273366,0.0485632310283938,-0.110139726828368]';
b = 1e6; 

row = size(cij,2);
% 同样对z3, p1, p2处理
x_input = [z1; z2; z3; p1; p2; qd; qd_dot; qd_ddot];
% x_input = [z1; z2; qd; qd_dot; qd_ddot];
h = zeros(row,1); 

W_F_dot = zeros(row,1);
W_Q_dot = zeros(row,1);
for j = 1:1:row
    h(j) = exp(-norm(x_input-cij(:,j))^2/(b^2));
    W_F_dot(j) = gamma_NN_F * (z2 * h(j) - eta_F  * W_F(j));
    W_Q_dot(j) = gamma_NN_Q * (z3 * h(j)- eta_Q  * W_Q(j));
    W_F_dot(j) = gamma_NN_F * (z2 * h(j) - eta_F * abs(z2) * W_F(j));
    W_Q_dot(j) = gamma_NN_Q * (z3 * h(j)- eta_Q * abs(z3) * W_Q(j));
%     W_F_dot(j) = Gamma_F(j,j) * (z2 * h(j) - eta_F  * W_F(j));
%     W_Q_dot(j) = Gamma_Q(j,j) * (z3 * h(j) - eta_Q  * W_Q(j));
    %限制幅值
    W_F_dot(j) = min(max(W_F_dot(j), -1000), 1000);
    W_Q_dot(j) = min(max(W_Q_dot(j), -1e-5), 1e-5);
end
%%
W_F_next = W_F_dot * ts + W_F;
W_Q_next = W_Q_dot * ts + W_Q;
%-------Output--------
RBFNN_F = W_F'*h;                                                               % 控制器输出电压
RBFNN_Q = W_Q'*h;  
% RBFNN_F = min(max(RBFNN_F, -100), 100);
% % RBFNN_Q = min(max(RBFNN_Q, -1e-5), 1e-4);
U_F = RBFNN_F*200;
U_Q = RBFNN_Q;
look  = h;

== matlab function RBFNN_1221/RBFNN_muti ==
  data: W_F input; W_Q input; U_F output; U_Q output; z1 input; z2 input; W_F_next output; W_Q_next output; W_F_dot output; z3 input; p1 input; p2 input; qd input; qd_dot input; qd_ddot input; gamma_NN_F input; gamma_NN_Q input; eta_F input; eta_Q input; look output
function [U_F, U_Q, W_F_next, W_Q_next, W_F_dot, look] = RBFNN(W_F, W_Q, z1, z2, z3, p1, p2, qd, qd_dot, qd_ddot, gamma_NN_F, gamma_NN_Q, eta_F, eta_Q)

% 仿真环境
ts = 0.0002;

%-------控制器需输入信息--------
num_joint = 2;
% RBFNN控制参数
%手腕关节中心点参数
cij_wrist= [-0.499106221625804,-0.499106221625804,2005.79872399738,2639144.26212096,2223202.48890840,-0.493324863755757,-0.0232163020531828,0.127650732846403;
            -1.12620134740565,-1.12620134740565,2952.38958819554,4234769.00352520,2070148.36236487,0.196658457787049,0.0133039268692362,-0.0826238790945131;
            -1.11695482722882,-1.11695482722882,3165.28189098781,3836085.68692222,1999734.92258975,0.153237256316932,0.0767773705194676,-0.369349406570774;
            -1.05951865103650,-1.05951865103650,3414.12364345425,3393273.20854046,2007071.20329101,-0.0589190714477196,0.00750783405961825,-0.229262334963137;
            -0.694285708154741,-0.694285708154741,2654.85166253362,2956383.72448738,2078438.60445473,-0.376420334916739,-0.0230368382437097,0.424736764481809;]';
b_wrist = 5e5;                                                                                          
%小臂关节宽度参数
cij_smallarm=[0.389378684114822,0.389378684114822,1114.48921420220,2616316.53671734,2561038.64169264,-1.51576839999243,0.0330866807450680,0.376260717223002;
              0.293961363490511,0.293961363490511,1376.96510708330,1983893.02565082,2835982.84668336,-1.00781767484497,0.0132794411754619,-0.158087018741097;
              0.246732699787306,0.246732699787306,1066.31436602314,2236325.53621658,2640181.79532095,-1.18241003990621,0.0473775864824768,-0.407578031102508;
              0.130205532666544,0.130205532666544,989.277438875963,3027371.69467571,2623425.14421574,-1.66183402604207,-0.118216514747365,0.309722684668361;
              0.0966671798383473,0.0966671798383473,813.586783016290,3422884.21291866,2722998.31843150,-1.69878574683684,-0.0124343039830796,0.0866126854764769]';
b_smallarm = 8e5;   
cij = zeros(8,5,num_joint);
cij(:,:,1) = cij_smallarm;  cij(:,:,2) = cij_wrist; 

b = [b_smallarm, b_wrist];
row = size(cij,2);
% 同样对z3, p1, p2处理
x_input = [z1, z2, z3, p1, p2, qd, qd_dot, qd_ddot]';
h = zeros(row,num_joint); 

W_F_dot = zeros(row,num_joint);
W_Q_dot = zeros(row,num_joint);
W_F_next = zeros(row,num_joint);
W_Q_next = zeros(row,num_joint);

for i = 1:num_joint  % 对每个自由度进行更新
    for j = 1:row  % 对每个RBF神经元进行更新
        h(j,i) = exp(-norm(x_input(:,i) - cij(:,j,i))^2 / (b(i)^2));  % 计算每个自由度的RBF响应
        W_F_dot(j,i) = gamma_NN_F(i) * (z2(i) * h(j,i) - eta_F(i) * abs(z2(i)) *W_F(j,i));
        W_Q_dot(j,i) = gamma_NN_Q(i) * (z3(i) * h(j,i) - eta_Q(i) * abs(z3(i)) * W_Q(j,i));
        %限制幅值
        W_F_dot(j,i) = min(max(W_F_dot(j,i), -1000), 1000);
        W_Q_dot(j,i) = min(max(W_Q_dot(j,i), -1e-5), 1e-5);
        W_F_next(j,i) = W_F_dot(j,i) * ts + W_F(j,i);
        W_Q_next(j,i) = W_Q_dot(j,i) * ts + W_Q(j,i);
    end
end

RBFNN_F = zeros(num_joint,1);
RBFNN_Q = zeros(num_joint,1);

%-------Output--------
for index = 1 : num_joint
    RBFNN_F(index) = W_F(:,index)'* h(:,index);                                                               % 控制器输出电压
    RBFNN_Q(index) = W_Q(:,index)'* h(:,index);  
end 
% RBFNN_F = min(max(RBFNN_F, -100), 100);
% % RBFNN_Q = min(max(RBFNN_Q, -1e-5), 1e-4);
U_F = RBFNN_F*200;
U_Q = RBFNN_Q;
look  = [0,0];

== matlab function RBFNN_1221/RBFNN_smallarm ==
  data: W_F input; W_Q input; U_F output; U_Q output; z1 input; z2 input; W_F_next output; W_Q_next output; W_F_dot output; z3 input; p1 input; p2 input; qd input; qd_dot input; qd_ddot input; gamma_NN_F input; gamma_NN_Q input; eta_F input; eta_Q input; look output
function [U_F, U_Q, W_F_next, W_Q_next, W_F_dot, look] = RBFNN(W_F, W_Q, z1, z2, z3, p1, p2, qd, qd_dot, qd_ddot, gamma_NN_F, gamma_NN_Q, eta_F, eta_Q)

% 仿真环境
ts = 0.0002;

%-------控制器需输入信息--------

% RBFNN控制参数

%手腕关节中心点参数
cij= [-0.499106221625804,-0.499106221625804,2005.79872399738,2639144.26212096,2223202.48890840,-0.493324863755757,-0.0232163020531828,0.127650732846403;
            -1.12620134740565,-1.12620134740565,2952.38958819554,4234769.00352520,2070148.36236487,0.196658457787049,0.0133039268692362,-0.0826238790945131;
            -1.11695482722882,-1.11695482722882,3165.28189098781,3836085.68692222,1999734.92258975,0.153237256316932,0.0767773705194676,-0.369349406570774;
            -1.05951865103650,-1.05951865103650,3414.12364345425,3393273.20854046,2007071.20329101,-0.0589190714477196,0.00750783405961825,-0.229262334963137;
            -0.694285708154741,-0.694285708154741,2654.85166253362,2956383.72448738,2078438.60445473,-0.376420334916739,-0.0230368382437097,0.424736764481809;]';
b = 5e5;                                                                                          
%小臂关节宽度参数
cij=[0.389378684114822,0.389378684114822,1114.48921420220,2616316.53671734,2561038.64169264,-1.51576839999243,0.0330866807450680,0.376260717223002;
              0.293961363490511,0.293961363490511,1376.96510708330,1983893.02565082,2835982.84668336,-1.00781767484497,0.0132794411754619,-0.158087018741097;
              0.246732699787306,0.246732699787306,1066.31436602314,2236325.53621658,2640181.79532095,-1.18241003990621,0.0473775864824768,-0.407578031102508;
              0.130205532666544,0.130205532666544,989.277438875963,3027371.69467571,2623425.14421574,-1.66183402604207,-0.118216514747365,0.309722684668361;
              0.0966671798383473,0.0966671798383473,813.586783016290,3422884.21291866,2722998.31843150,-1.69878574683684,-0.0124343039830796,0.0866126854764769]';
b = 8e5;   
% cij = zeros(8,5,2);
% cij(:,:,1) = cij_wrist; cij(:,:,2) = cij_smallarm;

row = size(cij,2);
% 同样对z3, p1, p2处理
x_input = [z1; z2; z3; p1; p2; qd; qd_dot; qd_ddot];
h = zeros(row,1); 

W_F_dot = zeros(row,1);
W_Q_dot = zeros(row,1);
for j = 1:1:row
    h(j) = exp(-norm(x_input-cij(:,j))^2/(b^2));
    W_F_dot(j) = gamma_NN_F * (z2 * h(j) - eta_F  * W_F(j));
    W_Q_dot(j) = gamma_NN_Q * (z3 * h(j)- eta_Q  * W_Q(j));
    W_F_dot(j) = gamma_NN_F * (z2 * h(j) - eta_F * abs(z2) * W_F(j));
    W_Q_dot(j) = gamma_NN_Q * (z3 * h(j)- eta_Q * abs(z3) * W_Q(j));
    %限制幅值
    W_F_dot(j) = min(max(W_F_dot(j), -1000), 1000);
    W_Q_dot(j) = min(max(W_Q_dot(j), -1e-5), 1e-5);
end




W_F_next = W_F_dot * ts + W_F;
W_Q_next = W_Q_dot * ts + W_Q;
%-------Output--------
RBFNN_F = W_F'*h;                                                               % 控制器输出电压
RBFNN_Q = W_Q'*h;  
% RBFNN_F = min(max(RBFNN_F, -100), 100);
% % RBFNN_Q = min(max(RBFNN_Q, -1e-5), 1e-4);
U_F = RBFNN_F*200;
U_Q = RBFNN_Q;
look  = W_F;
